simulink model "SPath"  (R2020a)
settings: Solver=VariableStepAuto  StartTime=0.0  StopTime=150  RelTol=1e-3
values from neighbouring files (symbols this model uses):
  b = 0.4    [Takeoff.m]
  body_rate_0 = [0;0;0]    [Takeoff.m]
  Boundaries = [B1;B2;B3]    [Takeoff.m]
  Euler_0 = [0;0;0]    [Takeoff.m]
  g = [0;0;-9.8]    [Takeoff.m]
  I_Drone = [0.3933,0.3933,0.76]    [Takeoff.m]
  I_Tank = CalItank(m_tank,0.4,0.1,0.4,i)    [Takeoff.m]
  J = 0.00062    [Takeoff.m]
  K = 0.074    [Takeoff.m]
  k_T = MaxMotorThrsut/(MaxRPM^2)    (= 6.99167657551e-06)    [Takeoff.m]
  k_Thrsut2Torque = 0.021    [Takeoff.m]
  l = 0.5    [Takeoff.m]
  L = sqrt((x2-x1)^2 + (y2-y1)^2)    [Takeoff.m]
  m = m_drone + m_tank*percent    (= 36)    [Takeoff.m]    (also in animation.m = T_V1toI*T_V2toV1*T_BtoV2)
  m_drone = 20    [Takeoff.m]
  m_tank = 16    [Takeoff.m]
  MaxThrust = 4*MaxMotorThrsut    (= 529.2)    [Takeoff.m]
  MaxTilt = 30*pi/180    (= 0.523598775598)    [Takeoff.m]
  MaxTorque_XY = (T2-T1)*(l/sqrt(2))    [Takeoff.m]
  MaxVolt = 48    [Takeoff.m]
  MaxYawRate = 100*pi/180    (= 1.74532925199)    [Takeoff.m]
  MaxZVel = 2    [Takeoff.m]
  percent = 1    [Takeoff.m]
  Px1 = 0.2    [Takeoff.m]
  Pz1 = 1    [Takeoff.m]
  Pz2 = 100    [Takeoff.m]
  R = 0.0062    [Takeoff.m]
  SafeZone = 1.0    (= 1)    [Takeoff.m]
  ts = 0.01    [Takeoff.m]
  WayPts = [[XYZ_0(1) XYZ_0(2) XYZ_0(3)] ... (first row only)    [Takeoff.m]
  XYZ_0 = [0;0;0]    [Takeoff.m]
undefined symbols (not defined in the file or in its folder): b_tank, d_drone, d_tank, DiscIntNeverNeededParam, FlyVel, h_tank, NWay, PD1, PD2, PI1, PI2, PP1, PP2, Sensor0Dir, ts_out, WayPtsYaw
libraries: simulink x26, vrlib x4, simulink_extras x2
(part 1 of 3)
settings Model: NumberOfSteps=10  Creator=blaze8871  LastModifiedBy=blaze8871
settings DataIOCC: SaveTime=off

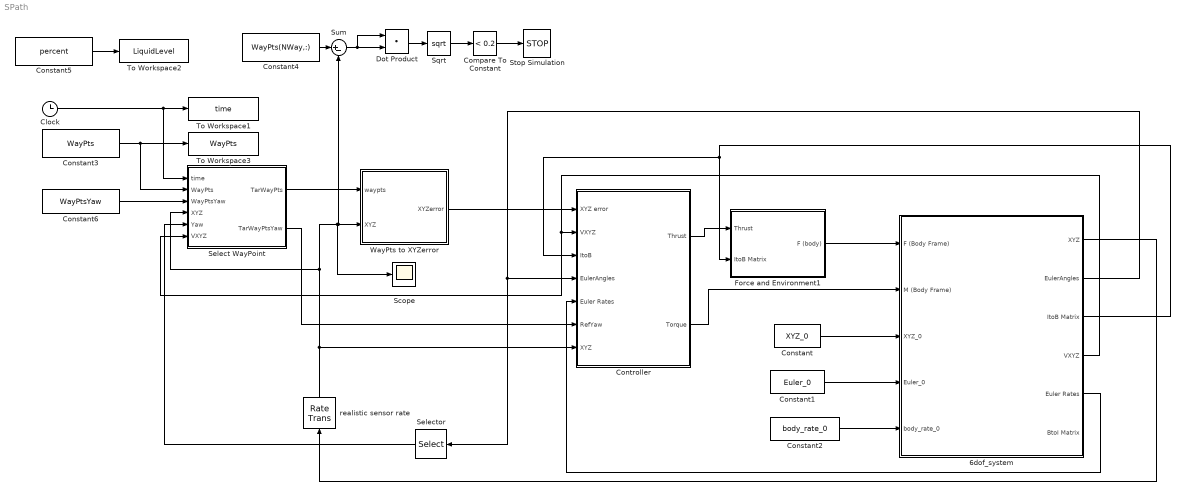
== system SPath ==
  6dof_system : Subsystem
  Clock : Clock
  Compare To Constant : simulink/Logic and Bit Operations/Compare To Constant  relop=<  const=0.2  OutDataTypeStr=boolean
  Constant : Constant  Value=XYZ_0  SampleTime=-1
  Constant1 : Constant  Value=Euler_0  SampleTime=-1
  Constant2 : Constant  Value=body_rate_0  SampleTime=-1
  Constant3 : Constant  Value=WayPts
  Constant4 : Constant  Value=WayPts(NWay,:)
  Constant5 : Constant  Value=percent
  Constant6 : Constant  Value=WayPtsYaw
  Controller : Subsystem
  Dot Product : DotProduct  InputSameDT=on  OutDataTypeStr=Inherit: Inherit via internal rule
  Force and Environment1 : Subsystem
  Scope : Scope
  Select WayPoint : Subsystem
  Selector : Selector  InputPortWidth=3  IndexOptions=Index vector (dialog)  Indices=[3]  OutputSizes=1
  Sqrt : Sqrt  SaturateOnIntegerOverflow=on
  Stop Simulation : Stop
  Sum : Sum  Inputs=|+-
  To Workspace1 : ToWorkspace  VariableName=time  SampleTime=ts_out
  To Workspace2 : ToWorkspace  VariableName=LiquidLevel  SampleTime=10000000
  To Workspace3 : ToWorkspace  VariableName=WayPts  SampleTime=10000000
  WayPts to XYZerror : MATLAB Function  TreatAsAtomicUnit=on
  realistic sensor rate : RateTransition  OutPortSampleTime=ts
  wires:
  Constant/1 -> 6dof_system/3(XYZ_0)
  Constant1/1 -> 6dof_system/4(Euler_0)
  Constant2/1 -> 6dof_system/5(body_rate_0)
  6dof_system/1(XYZ) -> realistic sensor rate/1
  6dof_system/2(EulerAngles) -> Selector/1, Controller/4(EulerAngles)
  WayPts to XYZerror/1(XYZerror) -> Controller/1(XYZ error)
  6dof_system/4(VXYZ) -> Select WayPoint/6(VXYZ), Controller/2(VXYZ)
  6dof_system/5(Euler Rates) -> Controller/5(Euler Rates)
  6dof_system/3(ItoB Matrix) -> Force and Environment1/2(ItoB Matrix), Controller/3(ItoB)
  Clock/1 -> To Workspace1/1, Select WayPoint/1(time)
  Constant3/1 -> Select WayPoint/2(WayPts), To Workspace3/1
  realistic sensor rate/1 -> WayPts to XYZerror/2(XYZ), Sum/2, Scope/1, Select WayPoint/4(XYZ), Controller/7(XYZ)
  Select WayPoint/1(TarWayPts) -> WayPts to XYZerror/1(waypts)
  Controller/1(Thrust) -> Force and Environment1/1(Thrust)
  Force and Environment1/1(F (body)) -> 6dof_system/1(F (Body Frame))
  Controller/2(Torque) -> 6dof_system/2(M (Body Frame))
  Constant6/1 -> Select WayPoint/3(WayPtsYaw)
  Select WayPoint/2(TarWayPtsYaw) -> Controller/6(RefYaw)
  Selector/1 -> Select WayPoint/5(Yaw)
  Constant4/1 -> Sum/1
  Sum/1 -> Dot Product/1, Dot Product/2
  Dot Product/1 -> Sqrt/1
  Sqrt/1 -> Compare To Constant/1
  Compare To Constant/1 -> Stop Simulation/1
  Constant5/1 -> To Workspace2/1

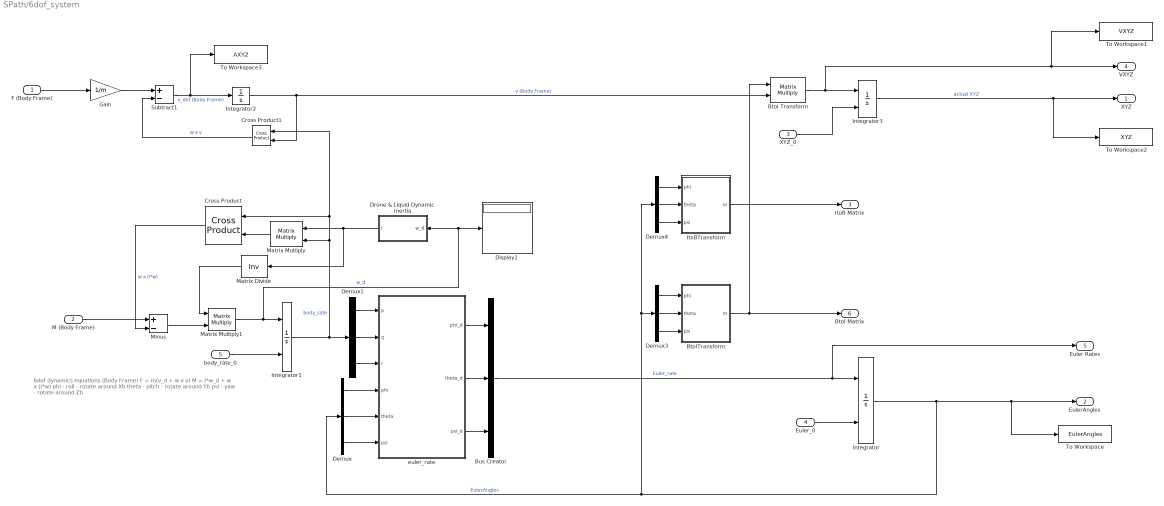
== system SPath/6dof_system ==
  note: 6dof dynamics equations
      | (Body Frame)
      |
      | F = m(v_d + w x v)
      | M = I*w_d + w x (I*w)
      |
      | phi - roll - rotate around Xb
      | theta - pitch - rotate around Yb
      | psi - yaw - rotate around Zb
  F (Body Frame) : Inport
  M (Body Frame) : Inport  Port=2
  XYZ_0 : Inport  Port=3
  Euler_0 : Inport  Port=4
  body_rate_0 : Inport  Port=5
  BtoI Transform : Product  Multiplication=Matrix(*)
  BtoITransform : MATLAB Function  TreatAsAtomicUnit=on
  Bus Creator : BusCreator  Inputs=3
  Cross Product : vrlib/Utilities/Cross Product
  Cross Product1 : vrlib/Utilities/Cross Product
  Demux{,1,3..4} (4 alike) : Demux  Outputs=3
  Display1 : Display
  Drone & Liquid Dynamic Inertia : Subsystem
  Gain : Gain  Gain=1/m
  Integrator : Integrator  InitialConditionSource=external  ContinuousStateAttributes='EulerAngle'
  Integrator1 : Integrator  InitialConditionSource=external  ContinuousStateAttributes='EulerAngle'
  Integrator2 : Integrator
  Integrator3 : Integrator  InitialConditionSource=external
  ItoBTransform : MATLAB Function  TreatAsAtomicUnit=on
  Matrix Divide : Product  Inputs=/  Multiplication=Matrix(*)
  Matrix Multiply : Product  Multiplication=Matrix(*)
  Matrix Multiply1 : Product  Multiplication=Matrix(*)
  Minus : Sum  Inputs=+-
  Subtract1 : Sum  Inputs=+-
  To Workspace : ToWorkspace  VariableName=EulerAngles  SampleTime=ts_out
  To Workspace1 : ToWorkspace  VariableName=VXYZ  SampleTime=ts_out
  To Workspace2 : ToWorkspace  VariableName=XYZ  SampleTime=ts_out
  To Workspace3 : ToWorkspace  VariableName=AXYZ  SampleTime=ts_out
  euler_rate : MATLAB Function  TreatAsAtomicUnit=on
  XYZ : Outport
  EulerAngles : Outport  Port=2
  ItoB Matrix : Outport  Port=3
  VXYZ : Outport  Port=4
  Euler Rates : Outport  Port=5
  BtoI Matrix : Outport  Port=6
  wires:
  F (Body Frame)/1 -> Gain/1
  Demux4/2 -> ItoBTransform/2(theta)
  euler_rate/1(phi_d) -> Bus Creator/1
  BtoITransform/1(m) -> BtoI Matrix/1, BtoI Transform/1
  Bus Creator/1 -> Euler Rates/1, Integrator/1  "Euler_rate"
  Matrix Multiply/1 -> Cross Product/2
  Demux3/2 -> BtoITransform/2(theta)
  Demux/2 -> euler_rate/5(theta)
  Demux4/1 -> ItoBTransform/1(phi)
  Subtract1/1 -> To Workspace3/1, Integrator2/1  "v_dot (Body Frame)"
  Cross Product1/1 -> Subtract1/2  "w x v"
  Demux1/1 -> euler_rate/1(p)
  Demux/3 -> euler_rate/6(psi)
  euler_rate/2(theta_d) -> Bus Creator/2
  Euler_0/1 -> Integrator/2
  Integrator3/1 -> To Workspace2/1, XYZ/1  "actual XYZ"
  Cross Product/1 -> Minus/2  "w x (I*w)"
  M (Body Frame)/1 -> Minus/1
  body_rate_0/1 -> Integrator1/2
  Demux3/3 -> BtoITransform/3(psi)
  euler_rate/3(psi_d) -> Bus Creator/3
  Demux4/3 -> ItoBTransform/3(psi)
  Gain/1 -> Subtract1/1
  Demux3/1 -> BtoITransform/1(phi)
  Demux1/3 -> euler_rate/3(r)
  XYZ_0/1 -> Integrator3/2
  Demux/1 -> euler_rate/4(phi)
  Integrator2/1 -> Cross Product1/2, BtoI Transform/2  "v (Body Frame)"
  Integrator1/1 -> Cross Product1/1, Cross Product/1, Matrix Multiply/2, Demux1/1  "body_rate"
  Demux1/2 -> euler_rate/2(q)
  ItoBTransform/1(m) -> ItoB Matrix/1
  BtoI Transform/1 -> To Workspace1/1, VXYZ/1, Integrator3/1
  Minus/1 -> Matrix Multiply1/2
  Matrix Multiply1/1 -> Integrator1/1, Display1/1, Drone & Liquid Dynamic Inertia/1(w_d)  "w_d"
  Integrator/1 -> To Workspace/1, EulerAngles/1, Demux4/1, Demux3/1, Demux/1  "EulerAngles"
  Drone & Liquid Dynamic Inertia/1(I) -> Matrix Divide/1, Matrix Multiply/1
  Matrix Divide/1 -> Matrix Multiply1/1

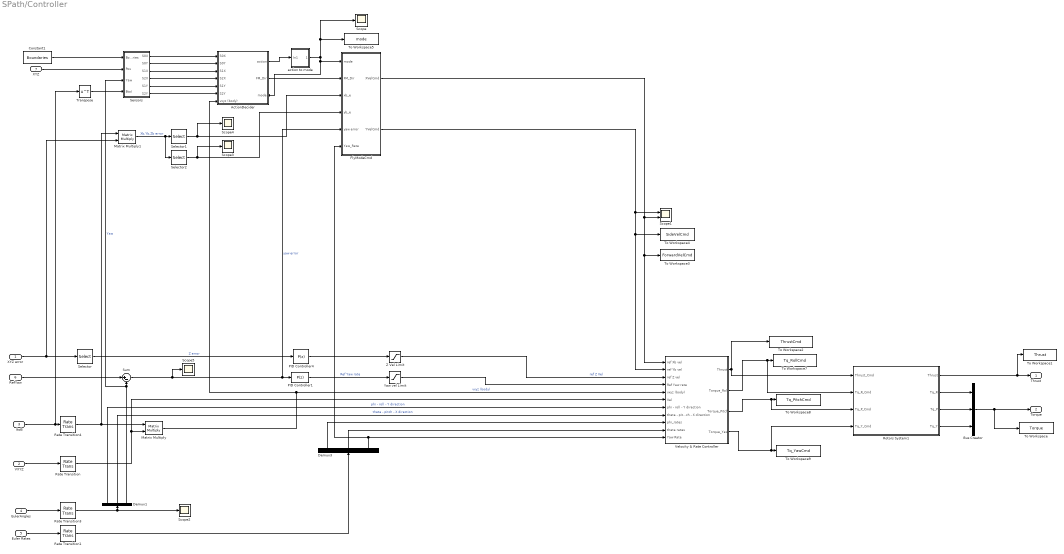
== system SPath/Controller ==
  XYZ error : Inport
  VXYZ : Inport  Port=2
  ItoB : Inport  Port=3
  EulerAngles : Inport  Port=4
  Euler Rates : Inport  Port=5
  RefYaw : Inport  Port=6
  XYZ : Inport  Port=7
  ActionDecider : Subsystem
      settings: PortSchema="{\"entries\":[{\"content\":{\"sides\":[{\"content\":{\"connectorIds\":[\"In1\",\"In2\",\"In3\",\"In4\",\"In5\",\"In6\",\"In7\"]},\"type\":\"ConnectorPlacement.EquallySpacedRectSide\",\"uuid\":\"6528d73d-eeac-4984-b7d0-00fbe024315f\"},{\"content\":{\"connectorIds\":[\"Out1\",\"Out2\",\"In8\"],\"side\":\"RIGHT\"},\"type\":\"ConnectorPlacement.EquallySpacedRectSide\",\"uuid\":\"439e9ece-61b3-4961-a65c-31503b83d5ef\"},{\"content\":{\"connectorIds\":[],\"side\":\"TOP\"},\"type\":\"ConnectorPlacement.EquallySpacedRectSide\",\"uuid\":\"090e856c-ba4d-4bc9-8397-8e5b6abdcbf3\"}]},\"type\":\"ConnectorPlacement.EquallySpacedConnector\",\"uuid\":\"55b5d35f-1a2c-4502-8428-f3d6ddd73aa6\"}],\"packageUris\":[\"http://schema.mathworks.com/mf0/Connector/19700101\"],\"version\":\"1.0\"}"
  Bus Creator : BusCreator  Inputs=3
  Constant1 : Constant  Value=Boundaries
  Demux1 : Demux  Outputs=3
  Demux3 : Demux  Outputs=3
  FlyModeCmd : Subsystem
  Matrix Multiply : Product  Multiplication=Matrix(*)
  Matrix Multiply1 : Product  Multiplication=Matrix(*)
  PID Controller1 : simulink/Continuous/PID Controller  Controller=P  Form=Parallel  TimeDomain=Discrete-time  UseExternalTs=off  SampleTime=ts  IntegratorMethod=Forward Euler  FilterMethod=Forward Euler  ControllerParametersSource=internal  P=1  I=1  D=0  UseFilter=on  N=100  TunerSelectOption=Transfer Function Based (PID Tuner App)  InitialConditionSource=internal  InitialConditionForIntegrator=0  InitialConditionForFilter=0  DifferentiatorICPrevScaledInput=0  ExternalReset=none  TrackingMode=off  Kt=1  LimitOutput=off  UpperSaturationLimit=inf  LowerSaturationLimit=-inf  LinearizeAsGain=on  AntiWindupMode=none  Kb=1  POutMin=[]  POutMax=[]  IOutMin=[]  IOutMax=[]  DOutMin=[]  DOutMax=[]  NOutMin=[]  NOutMax=[]  SumOutMin=[]  SumOutMax=[]  SaturationOutMin=[]  SaturationOutMax=[]  PParamMin=[]  PParamMax=[]  IParamMin=[]  IParamMax=[]  DParamMin=[]  DParamMax=[]  NParamMin=[]  NParamMax=[]  KbParamMin=[]  KbParamMax=[]  KtParamMin=[]  KtParamMax=[]  KbOutMin=[]  KbOutMax=[]  KtOutMin=[]  KtOutMax=[]  IntegratorOutMin=[]  IntegratorOutMax=[]  FilterOutMin=[]  FilterOutMax=[]  SumI1OutMin=[]  SumI1OutMax=[]  SumI2OutMin=[]  SumI2OutMax=[]  SumI3OutMin=[]  SumI3OutMax=[]  SumI4OutMin=[]  SumI4OutMax=[]  SumDOutMin=[]  SumDOutMax=[]  DifferentiatorOutMin=[]  DifferentiatorOutMax=[]  FilterDiffOutCoefMin=[]  FilterDiffOutCoefMax=[]  ReciprocalOutMin=[]  ReciprocalOutMax=[]  SumDenOutMin=[]  SumDenOutMax=[]  SumNumOutMin=[]  SumNumOutMax=[]  DivideOutMin=[]  DivideOutMax=[]  UdiffTsProdOutMin=[]  UdiffTsProdOutMax=[]  NTsProdOutMin=[]  NTsProdOutMax=[]  UintegralTsProdOutMin=[]  UintegralTsProdOutMax=[]  UngainTsProdOutMin=[]  UngainTsProdOutMax=[]  IntegratorContinuousStateAttributes=''  IntegratorStateMustResolveToSignalObject=off  IntegratorRTWStateStorageClass=Auto  FilterContinuousStateAttributes=''  FilterStateMustResolveToSignalObject=off  FilterRTWStateStorageClass=Auto  ParallelPVariant=InternalParameters  IdealPVariant=Disabled  IVariant=Disabled  DVariant=Disabled  IntegratorVariant=Disabled  SatVariant=Disabled  AWVariant=Disabled  PCopyVariant=Disabled  TRVariant=Disabled  FdbkBlocksVariant=Forward  IdealPFdbkVariant=Disabled  SatFdbkVariant=Disabled  DerivativeFilterVariant=Disabled  NVariant=Disabled  NCopyVariant=Disabled_SignalSpec  FilterICVariant=Disabled  IntegratorICVariant=Disabled  ExternalResetVariant=Disabled  TRSumVariant=Passthrough  SumFdbkVariant=Disabled  SumVariant=Passthrough_P  TsampFilterVariant=InternalTs  TsampNgainVariant=Passthrough  TsampIntegralVariant=Disabled_SignalSpec
  PID Controller4 : simulink/Continuous/PID Controller  Controller=P  Form=Parallel  TimeDomain=Discrete-time  UseExternalTs=off  SampleTime=ts  IntegratorMethod=Forward Euler  FilterMethod=Forward Euler  ControllerParametersSource=internal  P=Pz1  I=1  D=0  UseFilter=on  N=100  TunerSelectOption=Transfer Function Based (PID Tuner App)  InitialConditionSource=internal  InitialConditionForIntegrator=0  InitialConditionForFilter=0  DifferentiatorICPrevScaledInput=0  ExternalReset=none  TrackingMode=off  Kt=1  LimitOutput=off  UpperSaturationLimit=inf  LowerSaturationLimit=-inf  LinearizeAsGain=on  AntiWindupMode=none  Kb=1  POutMin=[]  POutMax=[]  IOutMin=[]  IOutMax=[]  DOutMin=[]  DOutMax=[]  NOutMin=[]  NOutMax=[]  SumOutMin=[]  SumOutMax=[]  SaturationOutMin=[]  SaturationOutMax=[]  PParamMin=[]  PParamMax=[]  IParamMin=[]  IParamMax=[]  DParamMin=[]  DParamMax=[]  NParamMin=[]  NParamMax=[]  KbParamMin=[]  KbParamMax=[]  KtParamMin=[]  KtParamMax=[]  KbOutMin=[]  KbOutMax=[]  KtOutMin=[]  KtOutMax=[]  IntegratorOutMin=[]  IntegratorOutMax=[]  FilterOutMin=[]  FilterOutMax=[]  SumI1OutMin=[]  SumI1OutMax=[]  SumI2OutMin=[]  SumI2OutMax=[]  SumI3OutMin=[]  SumI3OutMax=[]  SumI4OutMin=[]  SumI4OutMax=[]  SumDOutMin=[]  SumDOutMax=[]  DifferentiatorOutMin=[]  DifferentiatorOutMax=[]  FilterDiffOutCoefMin=[]  FilterDiffOutCoefMax=[]  ReciprocalOutMin=[]  ReciprocalOutMax=[]  SumDenOutMin=[]  SumDenOutMax=[]  SumNumOutMin=[]  SumNumOutMax=[]  DivideOutMin=[]  DivideOutMax=[]  UdiffTsProdOutMin=[]  UdiffTsProdOutMax=[]  NTsProdOutMin=[]  NTsProdOutMax=[]  UintegralTsProdOutMin=[]  UintegralTsProdOutMax=[]  UngainTsProdOutMin=[]  UngainTsProdOutMax=[]  IntegratorContinuousStateAttributes=''  IntegratorStateMustResolveToSignalObject=off  IntegratorRTWStateStorageClass=Auto  FilterContinuousStateAttributes=''  FilterStateMustResolveToSignalObject=off  FilterRTWStateStorageClass=Auto  ParallelPVariant=InternalParameters  IdealPVariant=Disabled  IVariant=Disabled  DVariant=Disabled  IntegratorVariant=Disabled  SatVariant=Disabled  AWVariant=Disabled  PCopyVariant=Disabled  TRVariant=Disabled  FdbkBlocksVariant=Forward  IdealPFdbkVariant=Disabled  SatFdbkVariant=Disabled  DerivativeFilterVariant=Disabled  NVariant=Disabled  NCopyVariant=Disabled_SignalSpec  FilterICVariant=Disabled  IntegratorICVariant=Disabled  ExternalResetVariant=Disabled  TRSumVariant=Passthrough  SumFdbkVariant=Disabled  SumVariant=Passthrough_P  TsampFilterVariant=InternalTs  TsampNgainVariant=Passthrough  TsampIntegralVariant=Disabled_SignalSpec
  Rate Transition{,1,3..4} (4 alike) : RateTransition  OutPortSampleTime=ts
  Rotors System1 : Subsystem
  Scope{,2..5} (5 alike) : Scope
  Scope1 : Scope  NumInputPorts=2
  Selector : Selector  InputPortWidth=3  IndexOptions=Index vector (dialog)  Indices=[3]  OutputSizes=1
  Selector1 : Selector  InputPortWidth=3  IndexOptions=Index vector (dialog)  Indices=[1]  OutputSizes=1
  Selector2 : Selector  InputPortWidth=3  IndexOptions=Index vector (dialog)  Indices=[2]  OutputSizes=1
  Sensors : Subsystem
  Sum : Sum  Inputs=|+-
  To Workspace : ToWorkspace  VariableName=Torque  SampleTime=ts_out
  To Workspace1 : ToWorkspace  VariableName=Thrust  SampleTime=ts_out
  To Workspace2 : ToWorkspace  VariableName=ThrustCmd  SampleTime=ts_out
  To Workspace3 : ToWorkspace  VariableName=ForwardVelCmd  SampleTime=ts_out
  To Workspace4 : ToWorkspace  VariableName=SideVelCmd  SampleTime=ts_out
  To Workspace5 : ToWorkspace  VariableName=mode  SampleTime=ts_out
  To Workspace7 : ToWorkspace  VariableName=Tq_RollCmd  SampleTime=ts_out
  To Workspace8 : ToWorkspace  VariableName=Tq_PitchCmd  SampleTime=ts_out
  To Workspace9 : ToWorkspace  VariableName=Tq_YawCmd  SampleTime=ts_out
  Transpose : Math  Operator=transpose  SaturateOnIntegerOverflow=on
  Velocity & Rate Controller : Subsystem
  Yaw vel Limit : Saturate  UpperLimit=MaxYawRate  LowerLimit=-MaxYawRate
  Z Vel Limit : Saturate  UpperLimit=MaxZVel  LowerLimit=-MaxZVel
  action to mode : Subsystem
  Thrust : Outport
  Torque : Outport  Port=2
  wires:
  Bus Creator/1 -> To Workspace/1, Torque/1
  VXYZ/1 -> Rate Transition/1
  Selector/1 -> PID Controller4/1  "Z error"
  EulerAngles/1 -> Rate Transition3/1
  Demux1/3 -> Sensors/3(Yaw), Sum/2  "Yaw"
  Sum/1 -> Scope5/1, FlyModeCmd/5(yaw error), PID Controller1/1  "yaw error"
  ItoB/1 -> Transpose/1, Rate Transition4/1
  XYZ error/1 -> Selector/1, Matrix Multiply1/2
  Rate Transition3/1 -> Scope2/1, Demux1/1
  Rate Transition4/1 -> Matrix Multiply/1, Matrix Multiply1/1
  Euler Rates/1 -> Rate Transition1/1
  Rate Transition1/1 -> Demux3/1
  Rate Transition/1 -> Matrix Multiply/2, Velocity & Rate Controller/6(Vel)
  Matrix Multiply/1 -> ActionDecider/7(vxyz (body)), Velocity & Rate Controller/5(vxyz (body))  "vxyz (body)"
  PID Controller4/1 -> Z Vel Limit/1
  PID Controller1/1 -> Yaw vel Limit/1  "Ref Yaw rate"
  Demux1/1 -> Velocity & Rate Controller/7(phi - roll - Y direction)  "phi - roll - Y direction"
  Demux1/2 -> Velocity & Rate Controller/8(theta - pitch - X direction)  "theta - pitch - X direction"
  Demux3/1 -> Velocity & Rate Controller/9(phi_rates)
  Demux3/2 -> Velocity & Rate Controller/10(theta rates)
  Demux3/3 -> FlyModeCmd/6(Yaw_Rate), Velocity & Rate Controller/11(Yaw Rate)
  Yaw vel Limit/1 -> Velocity & Rate Controller/4(Ref Yaw rate)
  RefYaw/1 -> Sum/1
  Velocity & Rate Controller/1(Thrust) -> Rotors System1/1(Thrust_Cmd), To Workspace2/1
  Velocity & Rate Controller/2(Torque_Roll) -> Rotors System1/2(Tq_R_Cmd), To Workspace7/1
  Velocity & Rate Controller/3(Torque_Pitch) -> Rotors System1/3(Tq_P_Cmd), To Workspace8/1
  Velocity & Rate Controller/4(Torque_Yaw) -> Rotors System1/4(Tq_Y_Cmd), To Workspace9/1
  Z Vel Limit/1 -> Velocity & Rate Controller/3(ref Z vel)  "ref Z Vel"
  Matrix Multiply1/1 -> Selector2/1, Selector1/1  "Xb,Yb,Zb error"
  Selector1/1 -> FlyModeCmd/3(xb_e), Scope4/1
  XYZ/1 -> Sensors/2(Pos)
  Transpose/1 -> Sensors/4(BtoI)
  Constant1/1 -> Sensors/1(Boundaries)
  action to mode/1(mode) -> ActionDecider/8(mode), FlyModeCmd/1(mode), To Workspace5/1, Scope/1
  Sensors/1(S0X) -> ActionDecider/1(S0X)
  Sensors/2(S0Y) -> ActionDecider/2(S0Y)
  Sensors/3(S1X) -> ActionDecider/3(S1X)
  Sensors/4(S2X) -> ActionDecider/4(S2X)
  Sensors/5(S1Y) -> ActionDecider/5(S1Y)
  Sensors/6(S2Y) -> ActionDecider/6(S2Y)
  ActionDecider/1(action) -> action to mode/1(In1)
  FlyModeCmd/1(XVelCmd) -> Scope1/2, Velocity & Rate Controller/1(ref Xb vel), To Workspace3/1
  FlyModeCmd/2(YVelCmd) -> To Workspace4/1, Velocity & Rate Controller/2(ref Yb vel), Scope1/1
  ActionDecider/2(FM_Dir) -> FlyModeCmd/2(FM_Dir)
  Selector2/1 -> Scope3/1, FlyModeCmd/4(yb_e)
  Rotors System1/1(Thrust) -> To Workspace1/1, Thrust/1
  Rotors System1/2(Tq_R) -> Bus Creator/1
  Rotors System1/3(Tq_P) -> Bus Creator/2
  Rotors System1/4(Tq_Y) -> Bus Creator/3

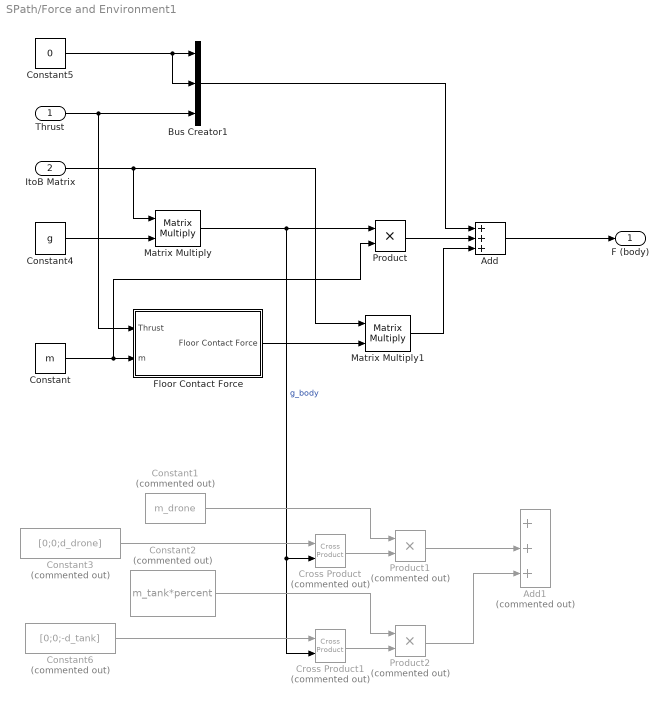
== system SPath/Force and Environment1 ==
  Thrust : Inport
  ItoB Matrix : Inport  Port=2
  Add : Sum  Inputs=+++
  Add1 : Sum  Commented=on  Inputs=+++
  Bus Creator1 : BusCreator  Inputs=3
  Constant : Constant  Value=m  SampleTime=ts
  Constant1 : Constant  Commented=on  Value=m_drone  SampleTime=ts
  Constant2 : Constant  Commented=on  Value=m_tank*percent  SampleTime=ts
  Constant3 : Constant  Commented=on  Value=[0;0;d_drone]  SampleTime=ts
  Constant4 : Constant  Value=g  SampleTime=-1
  Constant5 : Constant  Value=0  SampleTime=-1
  Constant6 : Constant  Commented=on  Value=[0;0;-d_tank]  SampleTime=ts
  Cross Product : vrlib/Utilities/Cross Product  Commented=on
  Cross Product1 : vrlib/Utilities/Cross Product  Commented=on
  Floor Contact Force : Subsystem
  Matrix Multiply : Product  Multiplication=Matrix(*)
  Matrix Multiply1 : Product  Multiplication=Matrix(*)
  Product : Product
  Product1 : Product  Commented=on
  Product2 : Product  Commented=on
  F (body) : Outport
  wires:
  Thrust/1 -> Floor Contact Force/1(Thrust), Bus Creator1/3
  ItoB Matrix/1 -> Matrix Multiply/1, Matrix Multiply1/1
  Constant5/1 -> Bus Creator1/2, Bus Creator1/1
  Add/1 -> F (body)/1
  Constant/1 -> Product/2, Floor Contact Force/2(m)
  Bus Creator1/1 -> Add/1
  Floor Contact Force/1(Floor Contact Force) -> Matrix Multiply1/2
  Matrix Multiply1/1 -> Add/3
  Constant4/1 -> Matrix Multiply/2
  Matrix Multiply/1 -> Cross Product/2, Cross Product1/2, Product/1  "g_body"
  Product/1 -> Add/2
  Constant3/1 -> Cross Product/1
  Cross Product/1 -> Product1/2
  Constant1/1 -> Product1/1
  Cross Product1/1 -> Product2/2
  Constant6/1 -> Cross Product1/1
  Constant2/1 -> Product2/1
  Product1/1 -> Add1/2
  Product2/1 -> Add1/3

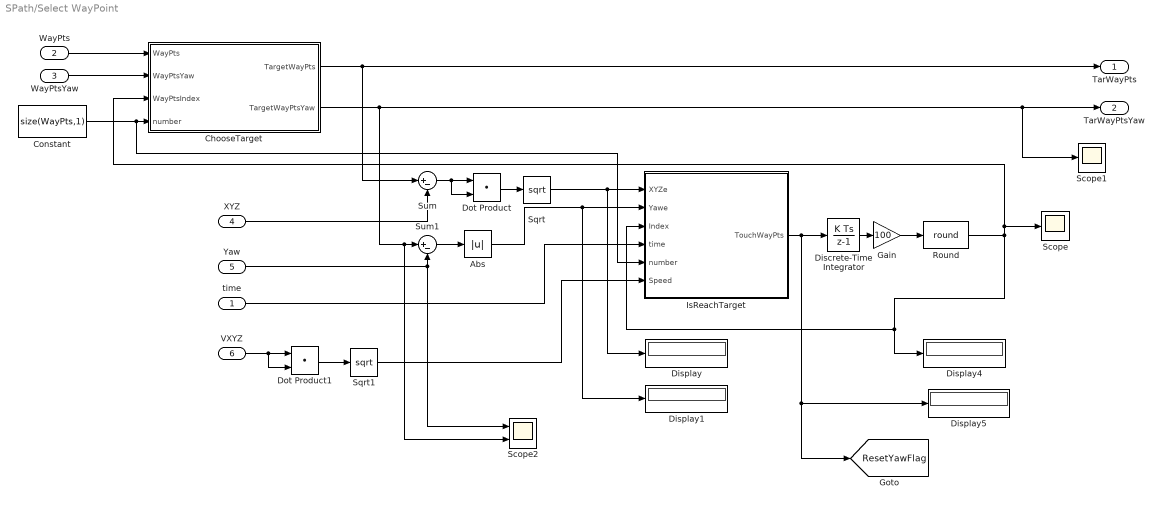
== system SPath/Select WayPoint ==
  time : Inport
  WayPts : Inport  Port=2
  WayPtsYaw : Inport  Port=3
  XYZ : Inport  Port=4
  Yaw : Inport  Port=5
  VXYZ : Inport  Port=6
  Abs : Abs
  ChooseTarget : MATLAB Function  TreatAsAtomicUnit=on
  Constant : Constant  Value=size(WayPts,1)
  Discrete-Time Integrator : DiscreteIntegrator  SampleTime=ts  ICPrevOutput=DiscIntNeverNeededParam  ICPrevScaledInput=DiscIntNeverNeededParam
  Display{,1,4..5} (4 alike) : Display
  Dot Product : DotProduct  InputSameDT=on  OutDataTypeStr=Inherit: Inherit via internal rule
  Dot Product1 : DotProduct  InputSameDT=on  OutDataTypeStr=Inherit: Inherit via internal rule
  Gain : Gain  Gain=100
  IsReachTarget : MATLAB Function  TreatAsAtomicUnit=on
  Round : Rounding  Operator=round
  Scope : Scope
  Scope1 : Scope
  Scope2 : Scope  NumInputPorts=2
  Sqrt : Sqrt  SaturateOnIntegerOverflow=on
  Sqrt1 : Sqrt  SaturateOnIntegerOverflow=on
  Sum : Sum  Inputs=|+-
  Sum1 : Sum  Inputs=|+-
  TarWayPts : Outport
  TarWayPtsYaw : Outport  Port=2
  tag scope: ResetYawFlag=global
  wires:
  WayPts/1 -> ChooseTarget/1(WayPts)
  ChooseTarget/1(TargetWayPts) -> Sum/1, TarWayPts/1
  Gain/1 -> Round/1
  IsReachTarget/1(TouchWayPts) -> [ResetYawFlag], Display5/1, Discrete-Time Integrator/1
  Discrete-Time Integrator/1 -> Gain/1
  time/1 -> IsReachTarget/4(time)
  WayPtsYaw/1 -> ChooseTarget/2(WayPtsYaw)
  ChooseTarget/2(TargetWayPtsYaw) -> Scope1/1, TarWayPtsYaw/1, Scope2/2, Sum1/1
  XYZ/1 -> Sum/2
  Sum/1 -> Dot Product/2, Dot Product/1
  Dot Product/1 -> Sqrt/1
  Sqrt/1 -> Display/1, IsReachTarget/1(XYZe)
  Yaw/1 -> Scope2/1, Sum1/2
  Sum1/1 -> Abs/1
  Abs/1 -> Display1/1, IsReachTarget/2(Yawe)
  Round/1 -> ChooseTarget/3(WayPtsIndex), Scope/1, Display4/1, IsReachTarget/3(Index)
  Constant/1 -> IsReachTarget/5(number), ChooseTarget/4(number)
  VXYZ/1 -> Dot Product1/2, Dot Product1/1
  Dot Product1/1 -> Sqrt1/1
  Sqrt1/1 -> IsReachTarget/6(Speed)

== system SPath/6dof_system/Drone & Liquid Dynamic Inertia ==
  w_d : Inport
  Constant : Constant  Value=I_Drone
  Constant1 : Constant  Value=I_Tank
  Constant2 : Constant  Value=m_tank
  Constant3 : Constant  Value=m_drone
  Constant4 : Constant  Value=d_drone
  Constant5 : Constant  Value=d_tank
  Constant6 : Constant  Commented=on  Value=h_tank
  Constant7 : Constant
  Display2 : Display
  DroneTankI : MATLAB Function  TreatAsAtomicUnit=on
  FullTankCR : MATLAB Function  Commented=on  TreatAsAtomicUnit=on
  Gain : Gain  Gain=percent
  Gain1 : Gain  Commented=on  Gain=percent
  Gain2 : Gain  Commented=on  Gain=1/b_tank
  MATLAB Function : MATLAB Function  Commented=on  TreatAsAtomicUnit=on
  Scope : Scope  Commented=on
  I : Outport
  wires:
  Constant/1 -> DroneTankI/1(I_D)
  w_d/1 -> FullTankCR/1(w_d)
  DroneTankI/1(I) -> Display2/1, I/1
  Constant1/1 -> DroneTankI/2(I_T)
  Constant3/1 -> DroneTankI/3(M_D)
  Gain/1 -> DroneTankI/4(M_T)
  Constant2/1 -> Gain/1
  Constant4/1 -> DroneTankI/5(Z_D)
  Constant5/1 -> DroneTankI/6(Z_T)
  Constant6/1 -> Gain1/1
  Gain1/1 -> Gain2/1
  Gain2/1 -> MATLAB Function/1(hb_ratio)
  MATLAB Function/1(C_R) -> Scope/1, FullTankCR/2(C_R)
  Constant7/1 -> DroneTankI/8(CR_Y), DroneTankI/7(CR_X)

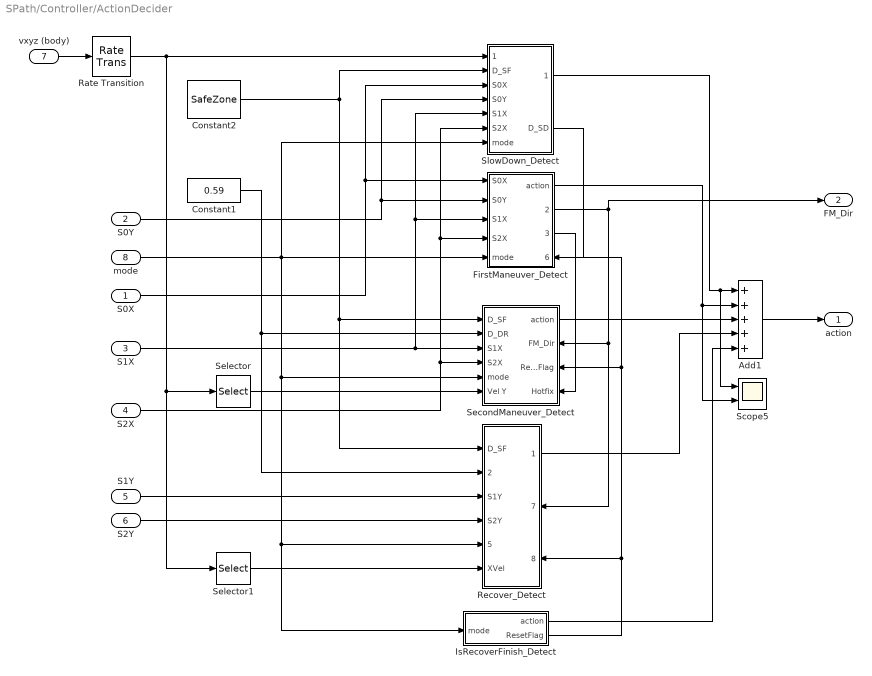
== system SPath/Controller/ActionDecider ==
  S0X : Inport
  S0Y : Inport  Port=2
  S1X : Inport  Port=3
  S2X : Inport  Port=4
  S1Y : Inport  Port=5
  S2Y : Inport  Port=6
  vxyz (body) : Inport  Port=7
  mode : Inport  Port=8
  Add1 : Sum  Inputs=+++++
  Constant1 : Constant  Value=0.59
  Constant2 : Constant  Value=SafeZone
  FirstManeuver_Detect : Subsystem
      settings: PortSchema="{\"entries\":[{\"content\":{\"sides\":[{\"content\":{\"connectorIds\":[\"In1\",\"In2\",\"In3\",\"In4\",\"In5\"]},\"type\":\"ConnectorPlacement.EquallySpacedRectSide\",\"uuid\":\"945ee97a-d82b-4fca-9f09-c45e443e0944\"},{\"content\":{\"connectorIds\":[\"Out1\",\"Out2\",\"Out3\",\"In6\"],\"side\":\"RIGHT\"},\"type\":\"ConnectorPlacement.EquallySpacedRectSide\",\"uuid\":\"4bd6b3d6-2281-48d2-b6b8-cb3bb3ed6829\"},{\"content\":{\"connectorIds\":[],\"side\":\"TOP\"},\"type\":\"ConnectorPlacement.EquallySpacedRectSide\",\"uuid\":\"51bde945-3930-4779-9c84-098ac5b13164\"}]},\"type\":\"ConnectorPlacement.EquallySpacedConnector\",\"uuid\":\"e3ef1a7a-d0e0-4983-b03e-2bd8c4580067\"}],\"packageUris\":[\"http://schema.mathworks.com/mf0/Connector/19700101\"],\"version\":\"1.0\"}"
  IsRecoverFinish_Detect : Subsystem
  Rate Transition : RateTransition  OutPortSampleTime=0.1
  Recover_Detect : Subsystem
      settings: PortSchema="{\"entries\":[{\"content\":{\"sides\":[{\"content\":{\"connectorIds\":[\"In1\",\"In2\",\"In3\",\"In4\",\"In5\",\"In6\"]},\"type\":\"ConnectorPlacement.EquallySpacedRectSide\",\"uuid\":\"2dac8849-fbab-4f90-b485-046e9f61bb72\"},{\"content\":{\"connectorIds\":[\"Out1\",\"In7\",\"In8\"],\"side\":\"RIGHT\"},\"type\":\"ConnectorPlacement.EquallySpacedRectSide\",\"uuid\":\"e2c3bd94-adb3-4689-a56c-030a8f3c429e\"},{\"content\":{\"connectorIds\":[],\"side\":\"TOP\"},\"type\":\"ConnectorPlacement.EquallySpacedRectSide\",\"uuid\":\"28962ba9-ba1d-4912-8fa5-5b5303f79a98\"}]},\"type\":\"ConnectorPlacement.EquallySpacedConnector\",\"uuid\":\"36001d2a-91a0-49e6-bdaa-b5fa5d0a07fa\"}],\"packageUris\":[\"http://schema.mathworks.com/mf0/Connector/19700101\"],\"version\":\"1.0\"}"
  Scope5 : Scope  NumInputPorts=2
  SecondManeuver_Detect : Subsystem
      settings: PortSchema="{\"entries\":[{\"content\":{\"sides\":[{\"content\":{\"connectorIds\":[\"In1\",\"In2\",\"In3\",\"In4\",\"In5\",\"In6\"]},\"type\":\"ConnectorPlacement.EquallySpacedRectSide\",\"uuid\":\"2dac8849-fbab-4f90-b485-046e9f61bb72\"},{\"content\":{\"connectorIds\":[\"Out1\",\"In7\",\"In8\",\"In9\"],\"side\":\"RIGHT\"},\"type\":\"ConnectorPlacement.EquallySpacedRectSide\",\"uuid\":\"e2c3bd94-adb3-4689-a56c-030a8f3c429e\"},{\"content\":{\"connectorIds\":[],\"side\":\"TOP\"},\"type\":\"ConnectorPlacement.EquallySpacedRectSide\",\"uuid\":\"28962ba9-ba1d-4912-8fa5-5b5303f79a98\"}]},\"type\":\"ConnectorPlacement.EquallySpacedConnector\",\"uuid\":\"36001d2a-91a0-49e6-bdaa-b5fa5d0a07fa\"}],\"packageUris\":[\"http://schema.mathworks.com/mf0/Connector/19700101\"],\"version\":\"1.0\"}"
  Selector : Selector  InputPortWidth=3  IndexOptions=Index vector (dialog)  Indices=[2]  OutputSizes=1
  Selector1 : Selector  InputPortWidth=3  IndexOptions=Index vector (dialog)  Indices=[1]  OutputSizes=1
  SlowDown_Detect : Subsystem
  action : Outport
  FM_Dir : Outport  Port=2
  wires:
  FirstManeuver_Detect/1(action) -> Add1/2, Scope5/2
  SlowDown_Detect/2(D_SD) -> ?
  IsRecoverFinish_Detect/1(action) -> Add1/5
  S2Y/1 -> Recover_Detect/4(S2Y)
  S1X/1 -> SlowDown_Detect/5(S1X), FirstManeuver_Detect/3(S1X), SecondManeuver_Detect/3(S1X)
  S0Y/1 -> SlowDown_Detect/4(S0Y), FirstManeuver_Detect/2(S0Y)
  Constant2/1 -> Recover_Detect/1(D_SF), SecondManeuver_Detect/1(D_SF), SlowDown_Detect/2(D_SF)
  SlowDown_Detect/1(action) -> Scope5/1, Add1/1
  FirstManeuver_Detect/2(FM_Dir) -> FM_Dir/1, Recover_Detect/7(FM_Dir), SecondManeuver_Detect/7(FM_Dir)
  Recover_Detect/1(action) -> Add1/4
  S0X/1 -> SlowDown_Detect/3(S0X), FirstManeuver_Detect/1(S0X)
  S1Y/1 -> Recover_Detect/3(S1Y)
  S2X/1 -> SlowDown_Detect/6(S2X), FirstManeuver_Detect/4(S2X), SecondManeuver_Detect/4(S2X)
  SecondManeuver_Detect/1(action) -> Add1/3
  Add1/1 -> action/1
  IsRecoverFinish_Detect/2(ResetFlag) -> FirstManeuver_Detect/6(ResetFlag), SecondManeuver_Detect/8(ResetFlag), Recover_Detect/8(ResetFlag)
  mode/1 -> IsRecoverFinish_Detect/1(mode), Recover_Detect/5(mode), SecondManeuver_Detect/5(mode), FirstManeuver_Detect/5(mode), SlowDown_Detect/7(mode)
  Constant1/1 -> SecondManeuver_Detect/2(D_DR), Recover_Detect/2(D_DR)
  Selector/1 -> SecondManeuver_Detect/6(Vel Y)
  vxyz (body)/1 -> Rate Transition/1
  Rate Transition/1 -> SlowDown_Detect/1(vxyz (body)), Selector/1, Selector1/1
  Selector1/1 -> Recover_Detect/6(XVel)
  FirstManeuver_Detect/3(HotFix) -> SecondManeuver_Detect/9(Hotfix)

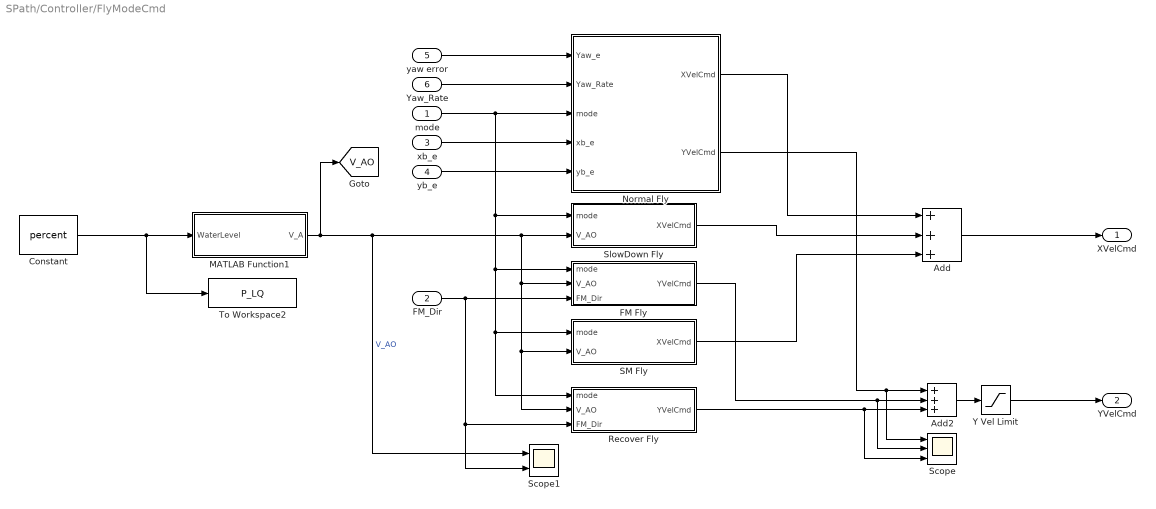
== system SPath/Controller/FlyModeCmd ==
  mode : Inport
  FM_Dir : Inport  Port=2
  xb_e : Inport  Port=3
  yb_e : Inport  Port=4
  yaw error : Inport  Port=5
  Yaw_Rate : Inport  Port=6
  Add : Sum  Inputs=+++
  Add2 : Sum  Inputs=+++
  Constant : Constant  Value=percent  SampleTime=ts_out
  FM Fly : MATLAB Function  TreatAsAtomicUnit=on
  MATLAB Function1 : MATLAB Function  TreatAsAtomicUnit=on
  Normal Fly : Subsystem
  Recover Fly : MATLAB Function  TreatAsAtomicUnit=on
  SM Fly : MATLAB Function  TreatAsAtomicUnit=on
  Scope : Scope  NumInputPorts=3
  Scope1 : Scope  NumInputPorts=2
  SlowDown Fly : MATLAB Function  TreatAsAtomicUnit=on
  To Workspace2 : ToWorkspace  VariableName=P_LQ  SampleTime=100000
  Y Vel Limit : Saturate  UpperLimit=5  LowerLimit=-5
  XVelCmd : Outport
  YVelCmd : Outport  Port=2
  tag scope: V_AO=global
  wires:
  Add/1 -> XVelCmd/1
  SlowDown Fly/1(XVelCmd) -> Add/2
  FM_Dir/1 -> Recover Fly/3(FM_Dir), Scope1/2, FM Fly/3(FM_Dir)
  mode/1 -> FM Fly/1(mode), SM Fly/1(mode), Recover Fly/1(mode), SlowDown Fly/1(mode), Normal Fly/3(mode)
  SM Fly/1(XVelCmd) -> Add/3
  Recover Fly/1(YVelCmd) -> Scope/3, Add2/3
  yaw error/1 -> Normal Fly/1(Yaw_e)
  Yaw_Rate/1 -> Normal Fly/2(Yaw_Rate)
  xb_e/1 -> Normal Fly/4(xb_e)
  yb_e/1 -> Normal Fly/5(yb_e)
  Normal Fly/1(XVelCmd) -> Add/1
  Normal Fly/2(YVelCmd) -> Scope/1, Add2/1
  Add2/1 -> Y Vel Limit/1
  Y Vel Limit/1 -> YVelCmd/1
  Constant/1 -> To Workspace2/1, MATLAB Function1/1(WaterLevel)
  MATLAB Function1/1(V_A) -> [V_AO], SlowDown Fly/2(V_AO), FM Fly/2(V_AO), Recover Fly/2(V_AO), SM Fly/2(V_AO), Scope1/1  "V_AO"
  FM Fly/1(YVelCmd) -> Scope/2, Add2/2

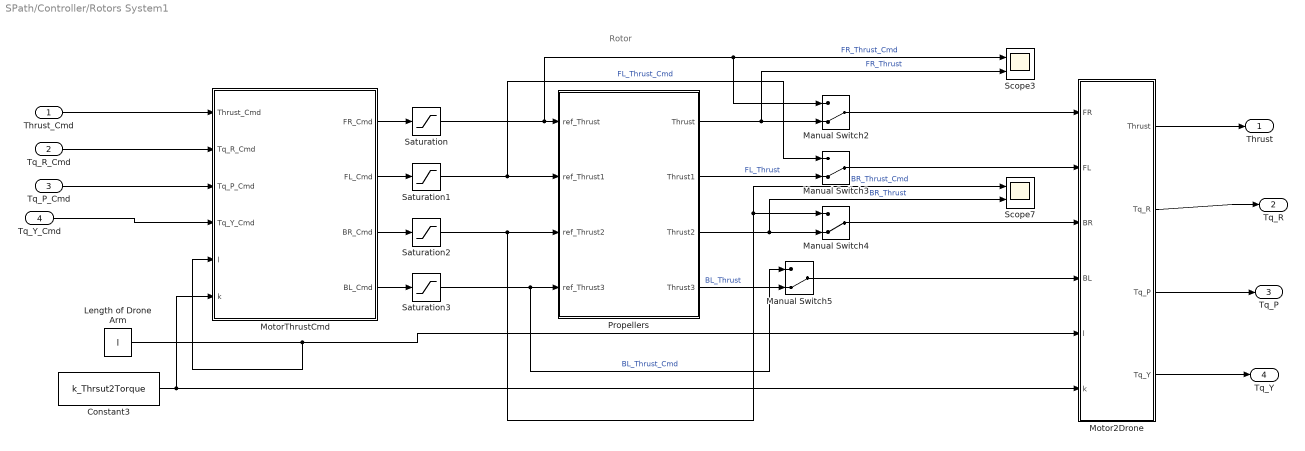
== system SPath/Controller/Rotors System1 ==
  note: Rotor
  Thrust_Cmd : Inport
  Tq_R_Cmd : Inport  Port=2
  Tq_P_Cmd : Inport  Port=3
  Tq_Y_Cmd : Inport  Port=4
  Constant3 : Constant  Value=k_Thrsut2Torque
  Length of Drone Arm : Constant  Value=l
  Manual Switch{2..5} (4 alike) : ManualSwitch  CurrentSetting=0
  Motor2Drone : MATLAB Function  TreatAsAtomicUnit=on
  MotorThrustCmd : MATLAB Function  TreatAsAtomicUnit=on
  Propellers : Subsystem
  Saturation{,1..3} (4 alike) : Saturate  UpperLimit=MaxThrust/4  LowerLimit=0
  Scope3 : Scope  NumInputPorts=2
  Scope7 : Scope  NumInputPorts=2
  Thrust : Outport
  Tq_R : Outport  Port=2
  Tq_P : Outport  Port=3
  Tq_Y : Outport  Port=4
  wires:
  Propellers/4(Thrust3) -> Manual Switch5/2  "BL_Thrust"
  Motor2Drone/4(Tq_Y) -> Tq_Y/1
  Propellers/3(Thrust2) -> Manual Switch4/2, Scope7/2  "BR_Thrust"
  Motor2Drone/2(Tq_R) -> Tq_R/1
  Saturation1/1 -> Manual Switch3/1, Propellers/2(ref_Thrust1)  "FL_Thrust_Cmd"
  Saturation3/1 -> Propellers/4(ref_Thrust3), Manual Switch5/1  "BL_Thrust_Cmd"
  Propellers/2(Thrust1) -> Manual Switch3/2  "FL_Thrust"
  MotorThrustCmd/2(FL_Cmd) -> Saturation1/1
  Constant3/1 -> MotorThrustCmd/6(k), Motor2Drone/6(k)
  MotorThrustCmd/4(BL_Cmd) -> Saturation3/1
  Saturation/1 -> Propellers/1(ref_Thrust), Scope3/1, Manual Switch2/1  "FR_Thrust_Cmd"
  Length of Drone Arm/1 -> Motor2Drone/5(l), MotorThrustCmd/5(l)
  Manual Switch2/1 -> Motor2Drone/1(FR)
  Motor2Drone/1(Thrust) -> Thrust/1
  MotorThrustCmd/1(FR_Cmd) -> Saturation/1
  Tq_P_Cmd/1 -> MotorThrustCmd/3(Tq_P_Cmd)
  Manual Switch5/1 -> Motor2Drone/4(BL)
  Propellers/1(Thrust) -> Manual Switch2/2, Scope3/2  "FR_Thrust"
  Tq_Y_Cmd/1 -> MotorThrustCmd/4(Tq_Y_Cmd)
  Manual Switch4/1 -> Motor2Drone/3(BR)
  Tq_R_Cmd/1 -> MotorThrustCmd/2(Tq_R_Cmd)
  Saturation2/1 -> Propellers/3(ref_Thrust2), Scope7/1, Manual Switch4/1  "BR_Thrust_Cmd"
  Thrust_Cmd/1 -> MotorThrustCmd/1(Thrust_Cmd)
  Motor2Drone/3(Tq_P) -> Tq_P/1
  Manual Switch3/1 -> Motor2Drone/2(FL)
  MotorThrustCmd/3(BR_Cmd) -> Saturation2/1

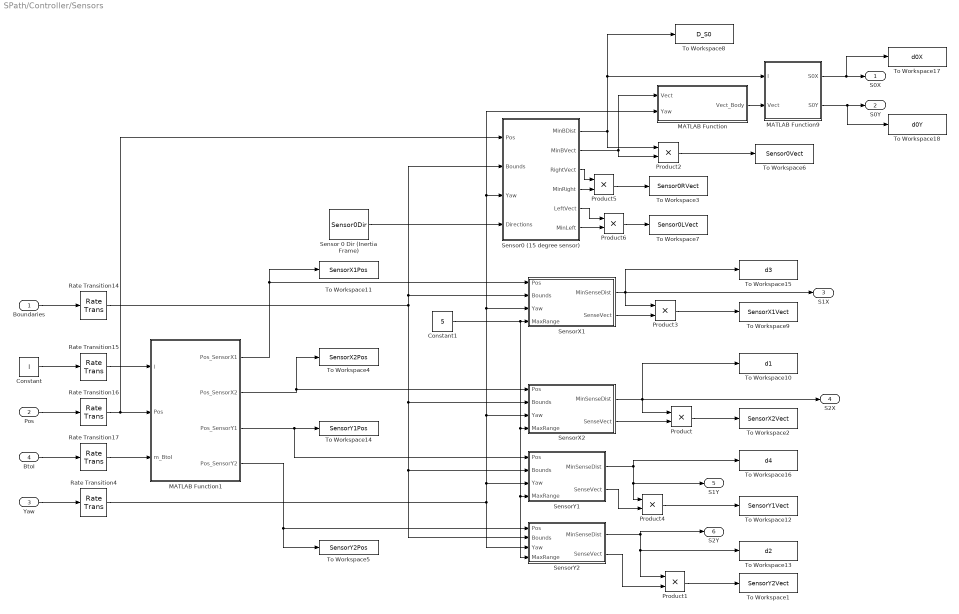
== system SPath/Controller/Sensors ==
  Boundaries : Inport
  Pos : Inport  Port=2
  Yaw : Inport  Port=3
  BtoI : Inport  Port=4
  Constant : Constant  Value=l
  Constant1 : Constant  Value=5
  MATLAB Function : MATLAB Function  TreatAsAtomicUnit=on
  MATLAB Function1 : MATLAB Function  TreatAsAtomicUnit=on
  MATLAB Function9 : MATLAB Function  TreatAsAtomicUnit=on
  Product{,1..6} (7 alike) : Product
  Rate Transition{4,14..17} (5 alike) : RateTransition  OutPortSampleTime=0.1
  Sensor 0 Dir (Inertia Frame) : Constant  Value=Sensor0Dir
  Sensor0 (15 degree sensor) : MATLAB Function  TreatAsAtomicUnit=on
  SensorX1 : MATLAB Function  TreatAsAtomicUnit=on
  SensorX2 : MATLAB Function  TreatAsAtomicUnit=on
  SensorY1 : MATLAB Function  TreatAsAtomicUnit=on
  SensorY2 : MATLAB Function  TreatAsAtomicUnit=on
  To Workspace1 : ToWorkspace  VariableName=SensorY2Vect  SampleTime=-1
  To Workspace10 : ToWorkspace  VariableName=d1  SampleTime=-1
  To Workspace11 : ToWorkspace  VariableName=SensorX1Pos  SampleTime=-1
  To Workspace12 : ToWorkspace  VariableName=SensorY1Vect  SampleTime=-1
  To Workspace13 : ToWorkspace  VariableName=d2  SampleTime=-1
  To Workspace14 : ToWorkspace  VariableName=SensorY1Pos  SampleTime=-1
  To Workspace15 : ToWorkspace  VariableName=d3  SampleTime=-1
  To Workspace16 : ToWorkspace  VariableName=d4  SampleTime=-1
  To Workspace17 : ToWorkspace  VariableName=d0X  SampleTime=-1
  To Workspace18 : ToWorkspace  VariableName=d0Y  SampleTime=-1
  To Workspace2 : ToWorkspace  VariableName=SensorX2Vect  SampleTime=-1
  To Workspace3 : ToWorkspace  VariableName=Sensor0RVect  SampleTime=-1
  To Workspace4 : ToWorkspace  VariableName=SensorX2Pos  SampleTime=-1
  To Workspace5 : ToWorkspace  VariableName=SensorY2Pos  SampleTime=-1
  To Workspace6 : ToWorkspace  VariableName=Sensor0Vect  SampleTime=-1
  To Workspace7 : ToWorkspace  VariableName=Sensor0LVect  SampleTime=-1
  To Workspace8 : ToWorkspace  VariableName=D_S0  SampleTime=-1
  To Workspace9 : ToWorkspace  VariableName=SensorX1Vect  SampleTime=-1
  S0X : Outport
  S0Y : Outport  Port=2
  S1X : Outport  Port=3
  S2X : Outport  Port=4
  S1Y : Outport  Port=5
  S2Y : Outport  Port=6
  wires:
  Boundaries/1 -> Rate Transition14/1
  Yaw/1 -> Rate Transition4/1
  Pos/1 -> Rate Transition16/1
  Constant/1 -> Rate Transition15/1
  BtoI/1 -> Rate Transition17/1
  MATLAB Function1/2(Pos_SensorX2) -> SensorX2/1(Pos), To Workspace4/1
  MATLAB Function1/4(Pos_SensorY2) -> To Workspace5/1, SensorY2/1(Pos)
  Sensor 0 Dir (Inertia Frame)/1 -> Sensor0 (15 degree sensor)/4(Directions)
  MATLAB Function1/1(Pos_SensorX1) -> SensorX1/1(Pos), To Workspace11/1
  MATLAB Function1/3(Pos_SensorY1) -> To Workspace14/1, SensorY1/1(Pos)
  Sensor0 (15 degree sensor)/1(MinBDist) -> Product2/1, To Workspace8/1, MATLAB Function9/1(l)
  Sensor0 (15 degree sensor)/2(MinBVect) -> Product2/2, MATLAB Function/1(Vect)
  SensorX2/2(SenseVect) -> Product/2
  SensorX2/1(MinSenseDist) -> To Workspace10/1, S2X/1, Product/1
  SensorX1/1(MinSenseDist) -> To Workspace15/1, Product3/1, S1X/1
  SensorX1/2(SenseVect) -> Product3/2
  SensorY1/1(MinSenseDist) -> S1Y/1, Product4/1, To Workspace16/1
  SensorY1/2(SenseVect) -> Product4/2
  SensorY2/1(MinSenseDist) -> S2Y/1, To Workspace13/1, Product1/1
  SensorY2/2(SenseVect) -> Product1/2
  Rate Transition14/1 -> Sensor0 (15 degree sensor)/2(Bounds), SensorX1/2(Bounds), SensorY2/2(Bounds), SensorY1/2(Bounds), SensorX2/2(Bounds)
  Rate Transition15/1 -> MATLAB Function1/1(l)
  Rate Transition16/1 -> Sensor0 (15 degree sensor)/1(Pos), MATLAB Function1/2(Pos)
  Rate Transition17/1 -> MATLAB Function1/3(m_BtoI)
  Rate Transition4/1 -> MATLAB Function/2(Yaw), Sensor0 (15 degree sensor)/3(Yaw), SensorX1/3(Yaw), SensorX2/3(Yaw), SensorY1/3(Yaw), SensorY2/3(Yaw)
  MATLAB Function9/1(S0X) -> To Workspace17/1, S0X/1
  MATLAB Function9/2(S0Y) -> To Workspace18/1, S0Y/1
  MATLAB Function/1(Vect_Body) -> MATLAB Function9/2(Vect)
  Product3/1 -> To Workspace9/1
  Product/1 -> To Workspace2/1
  Product4/1 -> To Workspace12/1
  Product1/1 -> To Workspace1/1
  Sensor0 (15 degree sensor)/3(RightVect) -> Product5/1
  Product2/1 -> To Workspace6/1
  Product5/1 -> To Workspace3/1
  Product6/1 -> To Workspace7/1
  Constant1/1 -> SensorY2/4(MaxRange), SensorY1/4(MaxRange), SensorX2/4(MaxRange), SensorX1/4(MaxRange)
  Sensor0 (15 degree sensor)/4(MinRight) -> Product5/2
  Sensor0 (15 degree sensor)/5(LeftVect) -> Product6/1
  Sensor0 (15 degree sensor)/6(MinLeft) -> Product6/2

== system SPath/Controller/Velocity & Rate Controller ==
  ref Xb vel : Inport
  ref Yb vel : Inport  Port=2
  ref Z vel : Inport  Port=3
  Ref Yaw rate : Inport  Port=4
  vxyz (body) : Inport  Port=5
  Vel : Inport  Port=6
  phi - roll - Y direction : Inport  Port=7
  theta - pitch - X direction : Inport  Port=8
  phi_rates : Inport  Port=9
  theta rates : Inport  Port=10
  Yaw Rate : Inport  Port=11
  Forward Velocity Controller : Subsystem
  Yaw Rate Controller : Subsystem
  Yb vel Controller : Subsystem
  Z vel Controller : Subsystem
  Thrust : Outport
  Torque_Roll : Outport  Port=2
  Torque_Pitch : Outport  Port=3
  Torque_Yaw : Outport  Port=4
  wires:
  Yb vel Controller/1(Torque_Roll) -> Torque_Roll/1
  Forward Velocity Controller/1(Torque_Pitch) -> Torque_Pitch/1
  theta - pitch - X direction/1 -> Forward Velocity Controller/3(theta - pitch - X direction)
  Z vel Controller/1(Thrust) -> Thrust/1
  phi - roll - Y direction/1 -> Yb vel Controller/3(phi)
  Ref Yaw rate/1 -> Yaw Rate Controller/1(Ref Yaw rate)
  ref Z vel/1 -> Z vel Controller/1(ref Z vel)
  vxyz (body)/1 -> Yb vel Controller/2(vb_y), Forward Velocity Controller/2(vxyz (body))
  Vel/1 -> Z vel Controller/2(Vel)
  theta rates/1 -> Forward Velocity Controller/4(theta rates)
  phi_rates/1 -> Yb vel Controller/4(phi_rates)
  Yaw Rate/1 -> Yaw Rate Controller/2(Yaw Rate)
  ref Xb vel/1 -> Forward Velocity Controller/1(ref Xb vel)
  Yaw Rate Controller/1(Torque_Yaw) -> Torque_Yaw/1
  ref Yb vel/1 -> Yb vel Controller/1(Ref Vb_y)

== system SPath/Controller/action to mode ==
  In1 : Inport
  Discrete-Time Integrator : DiscreteIntegrator  SampleTime=0.1  ICPrevOutput=DiscIntNeverNeededParam  ICPrevScaledInput=DiscIntNeverNeededParam
  Gain : Gain  Gain=10
  Round : Rounding  Operator=round
  mode : Outport
  wires:
  Discrete-Time Integrator/1 -> Gain/1
  Gain/1 -> Round/1
  Round/1 -> mode/1
  In1/1 -> Discrete-Time Integrator/1

== system SPath/Force and Environment1/Floor Contact Force ==
  Thrust : Inport
  m : Inport  Port=2
  Compare To Constant : simulink/Logic and Bit Operations/Compare To Constant  relop=>  const=0  OutDataTypeStr=boolean
  Discrete-Time Integrator : DiscreteIntegrator  SampleTime=-1  LimitOutput=on  UpperSaturationLimit=1  ICPrevOutput=DiscIntNeverNeededParam  ICPrevScaledInput=DiscIntNeverNeededParam
  MATLAB Function : MATLAB Function  TreatAsAtomicUnit=on
  MATLAB Function1 : MATLAB Function  TreatAsAtomicUnit=on
  Rate Transition : RateTransition  OutPortSampleTime=ts
  Scope : Scope
  Floor Contact Force : Outport
  wires:
  Rate Transition/1 -> MATLAB Function/1(Thrust)
  Discrete-Time Integrator/1 -> Compare To Constant/1
  MATLAB Function/1(DetectTakeOff) -> Discrete-Time Integrator/1
  Compare To Constant/1 -> MATLAB Function1/1(IsTakeOff), Scope/1
  Thrust/1 -> MATLAB Function1/2(Thrust), Rate Transition/1
  m/1 -> MATLAB Function/2(m), MATLAB Function1/3(m)
  MATLAB Function1/1(N) -> Floor Contact Force/1

== system SPath/Controller/ActionDecider/FirstManeuver_Detect ==
  S0X : Inport
  S0Y : Inport  Port=2
  S1X : Inport  Port=3
  S2X : Inport  Port=4
  mode : Inport  Port=5
  ResetFlag : Inport  Port=6
  Compare To Zero : simulink/Logic and Bit Operations/Compare To Zero  relop=>  OutDataTypeStr=boolean
  Discrete-Time Integrator : DiscreteIntegrator  ExternalReset=either  SampleTime=0.1  ICPrevOutput=DiscIntNeverNeededParam  ICPrevScaledInput=DiscIntNeverNeededParam
  Discrete-Time Integrator1 : DiscreteIntegrator  ExternalReset=either  SampleTime=0.1  ICPrevOutput=DiscIntNeverNeededParam  ICPrevScaledInput=DiscIntNeverNeededParam
  Discrete-Time Integrator2 : DiscreteIntegrator  ExternalReset=either  SampleTime=0.1  ICPrevOutput=DiscIntNeverNeededParam  ICPrevScaledInput=DiscIntNeverNeededParam
  FM_Detect : MATLAB Function  TreatAsAtomicUnit=on
  Gain : Gain  Gain=10
  Robust_Design : MATLAB Function  TreatAsAtomicUnit=on
  Round : Rounding  Operator=round
  Saturation : Saturate  UpperLimit=1  LowerLimit=-1
  Scope : Scope
  Scope2 : Scope
  action : Outport
  FM_Dir : Outport  Port=2
  HotFix : Outport  Port=3
  wires:
  mode/1 -> FM_Detect/1(mode), Robust_Design/1(mode)
  S2X/1 -> FM_Detect/5(S2X)
  S1X/1 -> FM_Detect/4(S1X)
  S0X/1 -> FM_Detect/2(S0X)
  S0Y/1 -> FM_Detect/3(S0Y)
  FM_Detect/2(FM_Dir) -> Discrete-Time Integrator/1
  Discrete-Time Integrator/1 -> Gain/1
  Gain/1 -> Round/1
  Round/1 -> Saturation/1  "FM_Dir"
  ResetFlag/1 -> Discrete-Time Integrator2/2, Discrete-Time Integrator/2, Discrete-Time Integrator1/2
  Discrete-Time Integrator1/1 -> Compare To Zero/1
  FM_Detect/3(HotFix) -> Discrete-Time Integrator1/1
  Compare To Zero/1 -> HotFix/1, Scope2/1
  Robust_Design/1(count) -> Discrete-Time Integrator2/1
  Discrete-Time Integrator2/1 -> FM_Detect/6(timeM1)  "time of mode 1"
  FM_Detect/1(action) -> action/1
  Saturation/1 -> FM_Dir/1, Scope/1

== system SPath/Controller/ActionDecider/IsRecoverFinish_Detect ==
  mode : Inport
  Discrete-Time Integrator1 : DiscreteIntegrator  SampleTime=0.1  ICPrevOutput=DiscIntNeverNeededParam  ICPrevScaledInput=DiscIntNeverNeededParam
  Discrete-Time Integrator2 : DiscreteIntegrator  SampleTime=0.1  ICPrevOutput=DiscIntNeverNeededParam  ICPrevScaledInput=DiscIntNeverNeededParam
  MATLAB Function : MATLAB Function  TreatAsAtomicUnit=on
  MATLAB Function1 : MATLAB Function  TreatAsAtomicUnit=on
  MATLAB Function2 : MATLAB Function  TreatAsAtomicUnit=on
  Scope : Scope
  Scope1 : Scope
  action : Outport
  ResetFlag : Outport  Port=2
  wires:
  mode/1 -> MATLAB Function1/1(u), MATLAB Function/1(mode), MATLAB Function2/1(u)
  MATLAB Function2/1(y) -> Discrete-Time Integrator2/1
  Discrete-Time Integrator2/1 -> MATLAB Function/3(t_md4), Scope1/1  "time of mode 4"
  MATLAB Function/1(action) -> action/1
  MATLAB Function/2(ResetFlag) -> ResetFlag/1
  MATLAB Function1/1(y) -> Discrete-Time Integrator1/1
  Discrete-Time Integrator1/1 -> MATLAB Function/2(t_md2), Scope/1  "time of mode 2"

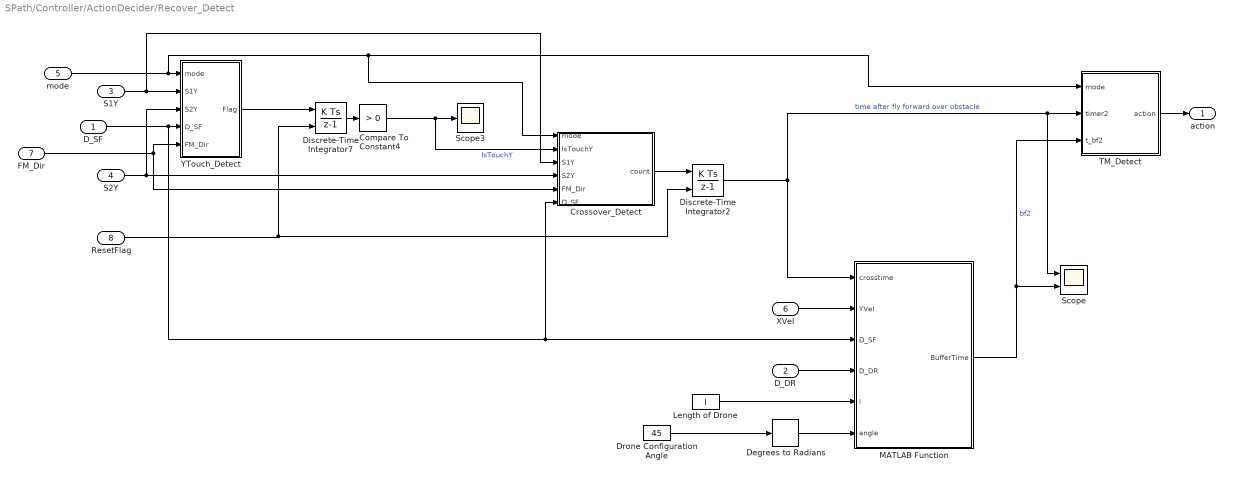
== system SPath/Controller/ActionDecider/Recover_Detect ==
  D_SF : Inport
  D_DR : Inport  Port=2
  S1Y : Inport  Port=3
  S2Y : Inport  Port=4
  mode : Inport  Port=5
  XVel : Inport  Port=6
  FM_Dir : Inport  Port=7
  ResetFlag : Inport  Port=8
  Compare To Constant4 : simulink/Logic and Bit Operations/Compare To Constant  relop=>  const=0  OutDataTypeStr=boolean
  Crossover_Detect : MATLAB Function  TreatAsAtomicUnit=on
  Degrees to Radians : simulink_extras/Transformations/Degrees to Radians
  Discrete-Time Integrator2 : DiscreteIntegrator  ExternalReset=either  SampleTime=0.1  ICPrevOutput=DiscIntNeverNeededParam  ICPrevScaledInput=DiscIntNeverNeededParam
  Discrete-Time Integrator7 : DiscreteIntegrator  ExternalReset=either  SampleTime=0.1  ICPrevOutput=DiscIntNeverNeededParam  ICPrevScaledInput=DiscIntNeverNeededParam
  Drone Configuration Angle : Constant  Value=45
  Length of Drone : Constant  Value=l
  MATLAB Function : MATLAB Function  TreatAsAtomicUnit=on
  Scope : Scope  NumInputPorts=2
  Scope3 : Scope
  TM_Detect : MATLAB Function  TreatAsAtomicUnit=on
  YTouch_Detect : MATLAB Function  TreatAsAtomicUnit=on
  action : Outport
  wires:
  S1Y/1 -> YTouch_Detect/2(S1Y), Crossover_Detect/3(S1Y)
  Compare To Constant4/1 -> Scope3/1, Crossover_Detect/2(IsTouchY)  "IsTouchY"
  S2Y/1 -> YTouch_Detect/3(S2Y), Crossover_Detect/4(S2Y)
  TM_Detect/1(action) -> action/1
  Crossover_Detect/1(count) -> Discrete-Time Integrator2/1
  Discrete-Time Integrator7/1 -> Compare To Constant4/1
  FM_Dir/1 -> YTouch_Detect/5(FM_Dir), Crossover_Detect/5(FM_Dir)
  YTouch_Detect/1(Flag) -> Discrete-Time Integrator7/1
  mode/1 -> YTouch_Detect/1(mode), Crossover_Detect/1(mode), TM_Detect/1(mode)
  D_SF/1 -> Crossover_Detect/6(D_SF), MATLAB Function/3(D_SF), YTouch_Detect/4(D_SF)
  ResetFlag/1 -> Discrete-Time Integrator7/2, Discrete-Time Integrator2/2
  Length of Drone/1 -> MATLAB Function/5(l)
  Degrees to Radians/1 -> MATLAB Function/6(angle)
  D_DR/1 -> MATLAB Function/4(D_DR)
  Drone Configuration Angle/1 -> Degrees to Radians/1
  XVel/1 -> MATLAB Function/2(YVel)
  Discrete-Time Integrator2/1 -> Scope/1, TM_Detect/2(timer2), MATLAB Function/1(crosstime)  "time after fly forward over obstacle"
  MATLAB Function/1(BufferTime) -> TM_Detect/3(t_bf2), Scope/2  "bf2"

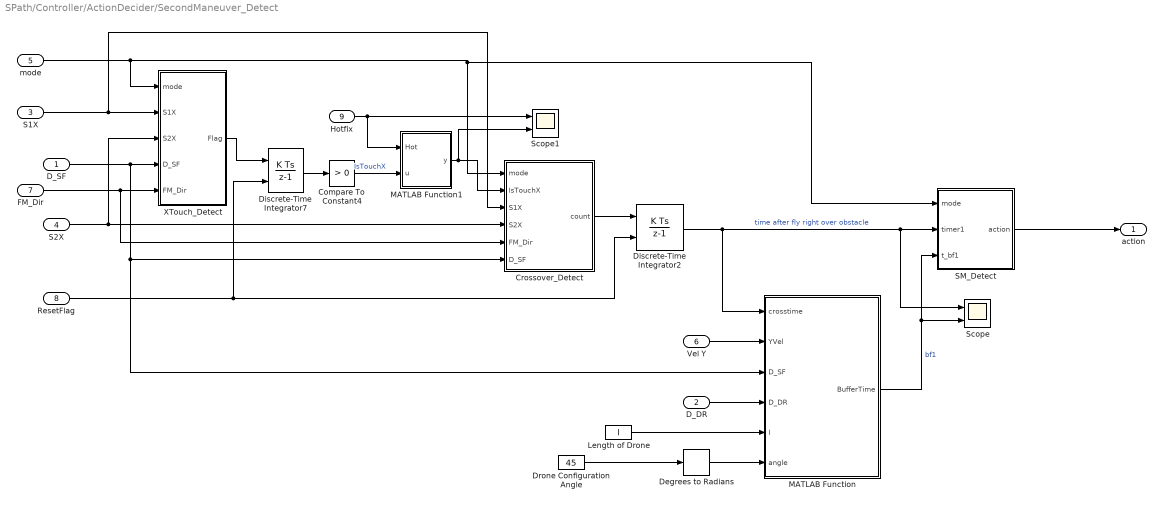
== system SPath/Controller/ActionDecider/SecondManeuver_Detect ==
  D_SF : Inport
  D_DR : Inport  Port=2
  S1X : Inport  Port=3
  S2X : Inport  Port=4
  mode : Inport  Port=5
  Vel Y : Inport  Port=6
  FM_Dir : Inport  Port=7
  ResetFlag : Inport  Port=8
  Hotfix : Inport  Port=9
  Compare To Constant4 : simulink/Logic and Bit Operations/Compare To Constant  relop=>  const=0  OutDataTypeStr=boolean
  Crossover_Detect : MATLAB Function  TreatAsAtomicUnit=on
  Degrees to Radians : simulink_extras/Transformations/Degrees to Radians
  Discrete-Time Integrator2 : DiscreteIntegrator  ExternalReset=either  SampleTime=0.1  ICPrevOutput=DiscIntNeverNeededParam  ICPrevScaledInput=DiscIntNeverNeededParam
  Discrete-Time Integrator7 : DiscreteIntegrator  ExternalReset=either  SampleTime=0.1  ICPrevOutput=DiscIntNeverNeededParam  ICPrevScaledInput=DiscIntNeverNeededParam
  Drone Configuration Angle : Constant  Value=45
  Length of Drone : Constant  Value=l
  MATLAB Function : MATLAB Function  TreatAsAtomicUnit=on
  MATLAB Function1 : MATLAB Function  TreatAsAtomicUnit=on
  SM_Detect : MATLAB Function  TreatAsAtomicUnit=on
  Scope : Scope  NumInputPorts=2
  Scope1 : Scope  NumInputPorts=2
  XTouch_Detect : MATLAB Function  TreatAsAtomicUnit=on
  action : Outport
  wires:
  Discrete-Time Integrator2/1 -> Scope/1, SM_Detect/2(timer1), MATLAB Function/1(crosstime)  "time after fly right over obstacle"
  MATLAB Function/1(BufferTime) -> Scope/2, SM_Detect/3(t_bf1)  "bf1"
  D_SF/1 -> Crossover_Detect/6(D_SF), MATLAB Function/3(D_SF), XTouch_Detect/4(D_SF)
  mode/1 -> XTouch_Detect/1(mode), Crossover_Detect/1(mode), SM_Detect/1(mode)
  XTouch_Detect/1(Flag) -> Discrete-Time Integrator7/1
  FM_Dir/1 -> Crossover_Detect/5(FM_Dir), XTouch_Detect/5(FM_Dir)
  Discrete-Time Integrator7/1 -> Compare To Constant4/1
  Crossover_Detect/1(count) -> Discrete-Time Integrator2/1
  SM_Detect/1(action) -> action/1
  S2X/1 -> Crossover_Detect/4(S2X), XTouch_Detect/3(S2X)
  S1X/1 -> Crossover_Detect/3(S1X), XTouch_Detect/2(S1X)
  ResetFlag/1 -> Discrete-Time Integrator7/2, Discrete-Time Integrator2/2
  Length of Drone/1 -> MATLAB Function/5(l)
  Drone Configuration Angle/1 -> Degrees to Radians/1
  Degrees to Radians/1 -> MATLAB Function/6(angle)
  D_DR/1 -> MATLAB Function/4(D_DR)
  Vel Y/1 -> MATLAB Function/2(YVel)
  Hotfix/1 -> MATLAB Function1/1(Hot), Scope1/1
  Compare To Constant4/1 -> MATLAB Function1/2(u)  "IsTouchX"
  MATLAB Function1/1(y) -> Scope1/2, Crossover_Detect/2(IsTouchX)

== system SPath/Controller/ActionDecider/SlowDown_Detect ==
  vxyz (body) : Inport
  D_SF : Inport  Port=2
  S0X : Inport  Port=3
  S0Y : Inport  Port=4
  S1X : Inport  Port=5
  S2X : Inport  Port=6
  mode : Inport  Port=7
  Constant4 : Constant  Value=MaxTilt
  Gain : Gain  Gain=1.2
  Gain1 : Gain  Gain=5
  MATLAB Function11 : MATLAB Function  TreatAsAtomicUnit=on
  MATLAB Function7 : MATLAB Function  TreatAsAtomicUnit=on
  Rate Transition5 : RateTransition  OutPortSampleTime=0.1
  Scope : Scope  NumInputPorts=3
  Selector2 : Selector  InputPortWidth=3  IndexOptions=Index vector (dialog)  Indices=[1]  OutputSizes=1
  SlowDown_Detect : MATLAB Function  TreatAsAtomicUnit=on
  Sum : Sum  Inputs=|++
  action : Outport
  D_SD : Outport  Port=2
  wires:
  Selector2/1 -> MATLAB Function7/2(Vx)
  D_SF/1 -> Gain1/1, SlowDown_Detect/3(D_SF)
  S0Y/1 -> SlowDown_Detect/5(S0Y), Scope/3
  S0X/1 -> Scope/1, SlowDown_Detect/4(S0X)
  vxyz (body)/1 -> Rate Transition5/1
  S1X/1 -> SlowDown_Detect/6(S1X)
  MATLAB Function11/1(y) -> MATLAB Function7/1(Accel)
  S2X/1 -> SlowDown_Detect/7(S2X)
  SlowDown_Detect/1(action) -> action/1
  MATLAB Function7/1(SlowDownDist) -> Gain/1
  mode/1 -> SlowDown_Detect/1(mode)
  Rate Transition5/1 -> Selector2/1
  Constant4/1 -> MATLAB Function11/1(u)
  Gain/1 -> Sum/1
  Sum/1 -> D_SD/1, Scope/2, SlowDown_Detect/2(D_SD)
  Gain1/1 -> Sum/2
